simulink model "task_2_1b"  (R2021b)
settings: Solver=VariableStepAuto  StartTime=0.0  StopTime=20  RelTol=1e-3
values from neighbouring files (symbols this model uses):
  k = 2.4716    [task_2_3.m]
  T = 0.0644    [task_2_3.m]
libraries: simulink x1
settings Model: Creator=osini  LastModifiedBy=osini

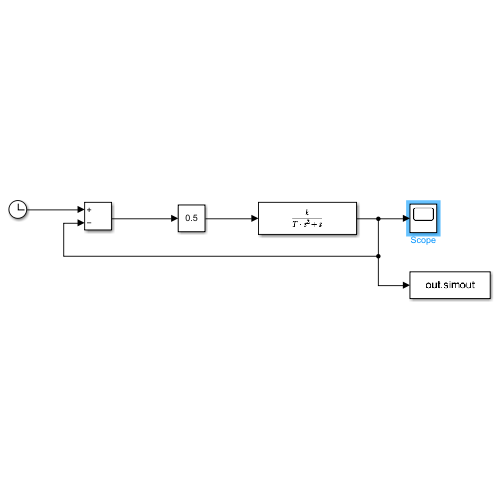
[thumbnail: Simulink's stored preview of the top-level diagram]
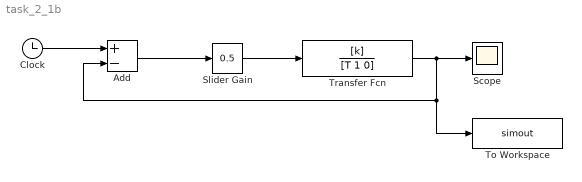
== system task_2_1b ==
  Add : Sum  Inputs=+-
  Clock : Clock
  Scope : Scope
  Slider Gain : simulink/Math Operations/Slider Gain  gain=0.5  low=0  high=1000
  To Workspace : ToWorkspace  VariableName=simout  SaveFormat=Timeseries  SampleTime=-1
  Transfer Fcn : TransferFcn  Numerator=[k]  Denominator=[T 1 0]
  wires:
  Add/1 -> Slider Gain/1
  Slider Gain/1 -> Transfer Fcn/1
  Transfer Fcn/1 -> To Workspace/1, Add/2, Scope/1
  Clock/1 -> Add/1
